simulink model "CQB_Mission_AdaptiveMod"  (R2024b)
settings: Solver=FixedStepAuto  StartTime=0.0  StopTime=210  FixedStep=1  RelTol=1e-3
settings Model: Creator=ARYA MGC  LastModifiedBy=ARYA MGC

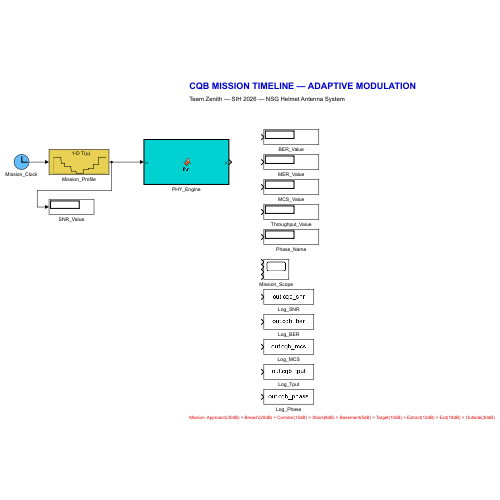
[thumbnail: Simulink's stored preview of the top-level diagram]
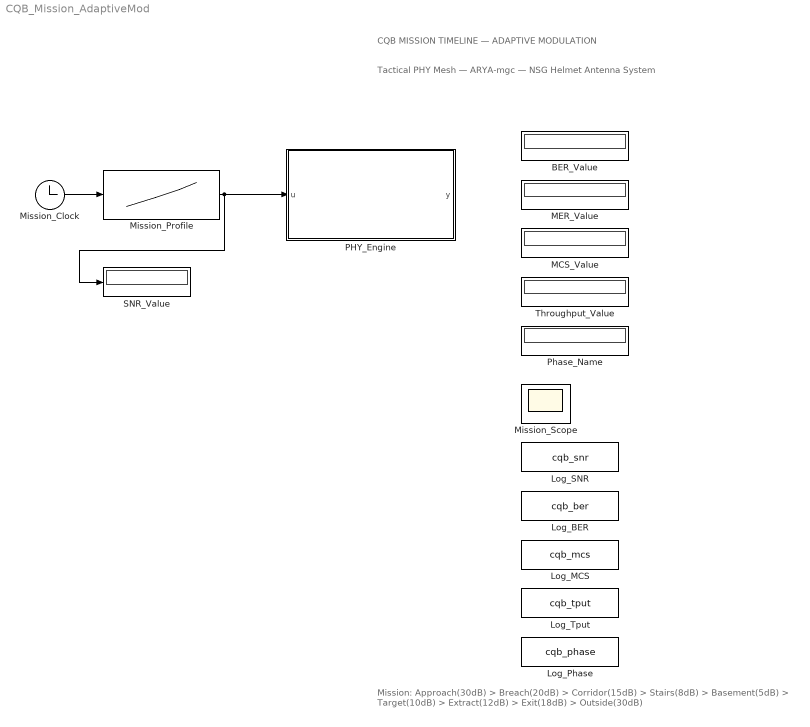
== system CQB_Mission_AdaptiveMod ==
  note: CQB MISSION TIMELINE — ADAPTIVE MODULATION
  note: Tactical PHY Mesh — ARYA-mgc — NSG Helmet Antenna System
  note: Mission: Approach(30dB) > Breach(20dB) > Corridor(15dB) > Stairs(8dB) > Basement(5dB) > Target(10dB) > Extract(12dB) > Exit(18dB) > Outside(30dB)
  BER_Value : Display
  Log_BER : ToWorkspace  VariableName=cqb_ber  SampleTime=-1
  Log_MCS : ToWorkspace  VariableName=cqb_mcs  SampleTime=-1
  Log_Phase : ToWorkspace  VariableName=cqb_phase  SampleTime=-1
  Log_SNR : ToWorkspace  VariableName=cqb_snr  SampleTime=-1
  Log_Tput : ToWorkspace  VariableName=cqb_tput  SampleTime=-1
  MCS_Value : Display
  MER_Value : Display
  Mission_Clock : Clock
  Mission_Profile : Lookup_n-D  NumberOfTableDimensions=1  BreakpointsForDimension1=[0 29 30 44 45 69 70 89 90 119 120 139 140 159 160 179 180 210]  Table="[30 30 20 20 15 15 8  8  5  5   10  10  12  12  18  18  30  30]"  InternalRulePriority=Speed  RndMeth=Simplest
  Mission_Scope : Scope  NumInputPorts=4
  PHY_Engine : MATLAB Function  TreatAsAtomicUnit=on
  Phase_Name : Display
  SNR_Value : Display
  Throughput_Value : Display
  wires:
  Mission_Clock/1 -> Mission_Profile/1
  Mission_Profile/1 -> PHY_Engine/1(u), SNR_Value/1

== matlab function CQB_Mission_AdaptiveMod/PHY_Engine ==
  data: u input; y output
function y = fcn(u)

y = u;
